simulink model "lsysid"  (Simulink 8.7)
settings: Solver=ode45  StartTime=0.0  StopTime=U(end,1)  RelTol=1e-3
values from neighbouring files (symbols this model uses):
  b = .5    (= 0.5)    [linid.m]
  h = 0.01    [Pendulum_linid.m]    (also in draw_pendulum.m = plot(0,0,'MarkerSize',20,'Marker','+','LineWidth',5); linid.m = 0.1; params.m)
  u0 = 0    [Pendulum_linid.m]
  x0 = [pi;0;0;0;0]    [Pendulum_linid.m]    (also in linid.m = [2;0])
settings Model: Creator=Dick  LastModifiedBy=Dick
settings DataIOCC: SignalLoggingSaveFormat=ModelDataLogs
settings OptimizationCC: BooleanDataType=off
settings DebuggingCC: SaveWithParameterizedLinksMsg=none  SignalResolutionControl=TryResolveAllWithWarning  MultiTaskDSMMsg=warning  MultiTaskCondExecSysMsg=none
settings HardwareCC: ProdBitPerPointer=64  ProdLargestAtomicFloat=Float  ProdIntDivRoundTo=Zero  ProdEndianess=LittleEndian  ProdWordSize=64  ProdHWDeviceType=Intel->x86-64 (Windows64)  TargetUnknown=on
settings GRTTargetCC: GeneratePreprocessorConditionals=Use local settings  CombineOutputUpdateFcns=off  GRTInterface=on

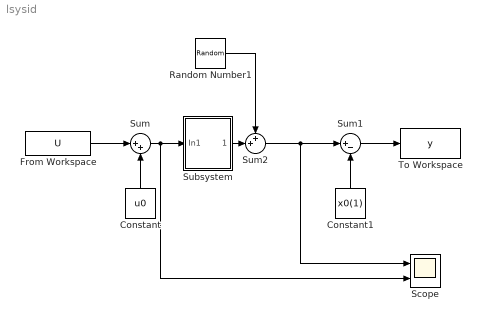
== system lsysid ==
  Constant : Constant  Value=u0
  Constant1 : Constant  Value=x0(1)
  From Workspace : FromWorkspace  VariableName=U  SampleTime=h
  Random Number1 : RandomNumber  Variance=1e-7  SampleTime=h
  Scope : Scope  NumInputPorts=2
  Subsystem : Subsystem
  Sum : Sum  Inputs=|++  SaturateOnIntegerOverflow=on  InputSameDT=on  OutDataTypeStr=Inherit: Same as first input
  Sum1 : Sum  Inputs=|+-  SaturateOnIntegerOverflow=on  InputSameDT=on  OutDataTypeStr=Inherit: Same as first input
  Sum2 : Sum  Inputs=++|  SaturateOnIntegerOverflow=on  InputSameDT=on  OutDataTypeStr=Inherit: Same as first input
  To Workspace : ToWorkspace  VariableName=y  SampleTime=h
  wires:
  From Workspace/1 -> Sum/1
  Sum/1 -> Subsystem/1(In1), Scope/2
  Constant/1 -> Sum/2
  Constant1/1 -> Sum1/2
  Sum1/1 -> To Workspace/1
  Sum2/1 -> Sum1/1, Scope/1
  Subsystem/1(Out1) -> Sum2/2
  Random Number1/1 -> Sum2/1

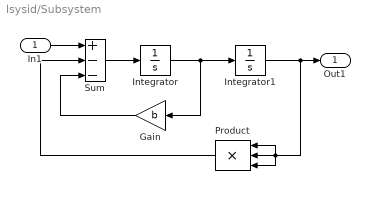
== system lsysid/Subsystem ==
  In1 : Inport
  Gain : Gain  Gain=b  SaturateOnIntegerOverflow=on  OutDataTypeStr=Inherit: Same as input  ParamDataTypeStr=Inherit: Same as input
  Integrator : Integrator  InitialCondition=x0(2)
  Integrator1 : Integrator  InitialCondition=x0(1)
  Product : Product  Inputs=3  SaturateOnIntegerOverflow=on  RndMeth=Zero  InputSameDT=on  OutDataTypeStr=Inherit: Same as first input
  Sum : Sum  Inputs=+--  SaturateOnIntegerOverflow=on  InputSameDT=on  OutDataTypeStr=Inherit: Same as first input
  Out1 : Outport
  wires:
  Integrator/1 -> Integrator1/1, Gain/1
  Sum/1 -> Integrator/1
  Integrator1/1 -> Product/2, Product/1, Product/3, Out1/1
  Product/1 -> Sum/2
  Gain/1 -> Sum/3
  In1/1 -> Sum/1
